simulink model "sim1"  (R2024a)
settings: Solver=FixedStepAuto  StartTime=0.0  StopTime=10.0  FixedStep=1e-3  RelTol=1e-3
settings Model: Creator=alexe  LastModifiedBy=alexe

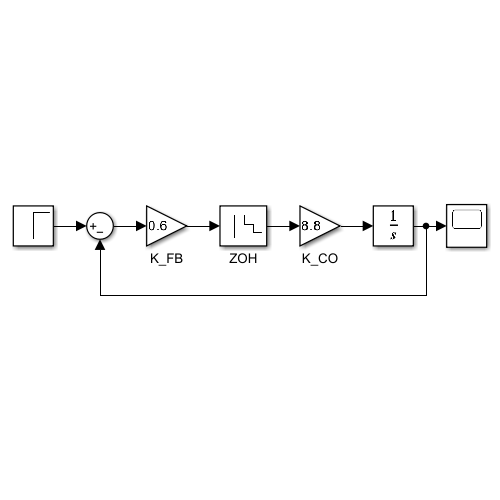
[thumbnail: Simulink's stored preview of the top-level diagram]
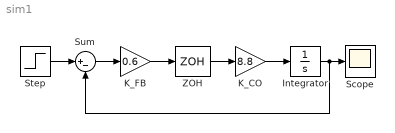
== system sim1 ==
  Integrator : Integrator
  K_CO : Gain  Gain=8.8
  K_FB : Gain  Gain=0.6
  Scope : Scope
  Step : Step  Time=0  SampleTime=0
  Sum : Sum  Inputs=|+-
  ZOH : ZeroOrderHold  SampleTime=0.25
  wires:
  Sum/1 -> K_FB/1
  Step/1 -> Sum/1
  K_FB/1 -> ZOH/1
  ZOH/1 -> K_CO/1
  K_CO/1 -> Integrator/1
  Integrator/1 -> Sum/2, Scope/1
